simulink model "ur5_v4"  (R2018a)
settings: Solver=VariableStepAuto  StartTime=0.0  StopTime=100.0  MaxStep=2.0  RelTol=1e-3
undefined symbols (not defined in the file): X, Y, Z
libraries: sm_lib x73, nesl_utility x26
(part 3 of 3)

== matlab function ur5_v4/MATLAB Function ==
  data: q1 input; qdot1 input; qddot1 input; tau1 output; q2 input; qdot2 input; qddot2 input; q3 input; qdot3 input; tau2 output; tau3 output; tau4 output; tau5 output; tau6 output; qddot3 input; q4 input; qdot4 input; qddot4 input; q5 input; qdot5 input; qddot5 input; q6 input; qdot6 input; qddot6 input; t input
function [tau1,tau2,tau3,tau4,tau5,tau6] = inverseDynamicsController(q1, qdot1, qddot1, q2, qdot2, qddot2, q3, qdot3, qddot3,q4, qdot4, qddot4,q5, qdot5, qddot5,q6, qdot6, qddot6, t)
    %inverseDynamicsController CTC
    
%     r = 0.7; % m
% %     
% %     % define the gains
% %     kd = eye(6) * 100;
% %     kp = eye(6) * 100;
% % 
% %     % defining the theta vector
% %     q = [q1; q2; q3; q4; q5; q6];
% %     q(1) = mod(q(1),sign(q(1)) * 2*pi);
% %     q(2) = mod(q(2),sign(q(2)) * 2*pi);
% %     q(3) = mod(q(3),sign(q(3)) * 2*pi);
% %     q(4) = mod(q(4),sign(q(4)) * 2*pi);
% %     q(5) = mod(q(5),sign(q(5)) * 2*pi);
% %     q(6) = mod(q(6),sign(q(6)) * 2*pi);
% % 
% %     % defining the theta dot vector
% %     qdot = [qdot1; qdot2; qdot3; qdot4; qdot5; qdot6];
% %     
% %     G = computeG(q);
% %     M = computeM(q);
% %     C = computeC(q, qdot);
% %     
% %     xd = [r * cos(t);...
% %           r * sin(t);...
% %           0.5;...
% %           0;...
% %           0;...
% %           0;...
% %           ];
% %     xdotd = [-r * sin(t);...
% %              r * cos(t);...
% %              0;...
% %              0;...
% %              0;...
% %              0];
% %          
% %     xddotd = [-r * cos(t);...
% %               -r * sin(t);...
% %               0;...
% %               0;...
% %               0;...
% %               0];
% %               
% %     mdl_ur5
% theta = [q1;q2;q3;q4;q5;q6];
% dtheta = [qdot1;qdot2;qdot3;qdot4;qdot5;qdot6];
% %% Dynamics
% Mmat = [ 0.826179504375*cos(2.0*t2 + t3) - 0.0565404972*sin(2.0*t2 + t3) + 1.20557253125*cos(2.0*t2) + 0.0000000000000000019573801614355403439437524183897*cos(t2 + t3) + 0.000000000000000014511003174485468031141763691783*sin(t2 + t3) + 0.826179504375*cos(t3) + 0.000000000000000015722565581023132984666028219267*sin(t2) - 0.0565404972*sin(t3) + 0.374967577853955*cos(2.0*t2 + 2.0*t3) - 0.052183553004*sin(2.0*t2 + 2.0*t3) + 1.6498961438878783371962262793672,                                                    0.015983221960800000770298430129775*cos(t2 + t3) + 0.11849133304875000319532105772424*sin(t2 + t3) + 0.00000000000000010117780855539904452958870603611*cos(t3) + 0.12838449087500000346210694590899*sin(t2) - 0.0000000000000000069242138918179886397619225021053*sin(t3) + 0.00000000000000019510093541407624091515398576369,                           0.015983221960800000770298430129775*cos(t2 + t3) + 0.11849133304875000319532105772424*sin(t2 + t3) + 0.000000000000000050588904277699522264794353018057*cos(t3) - 0.0000000000000000034621069459089943198809612510527*sin(t3) + 0.000000000000000047460881260547746144125949805253;...
%                                                                                                                                   0.015983221960800000770298430129775*cos(t2 + t3) + 0.11849133304875000319532105772424*sin(t2 + t3) + 0.00000000000000010117780855539904452958870603611*cos(t3) + 0.12838449087500000346210694590899*sin(t2) - 0.0000000000000000069242138918179886397619225021053*sin(t3) + 0.00000000000000019510093541407624091515398576369, 3.0976769848028282159067604929052e-33*cos(2.0*t2 + t3) - 2.1199290948066343006048283768305e-34*sin(2.0*t2 + t3) + 4.5201729936265140290864586741331e-33*cos(2.0*t2) + 1.65235900875*cos(t3) - 0.1130809944*sin(t3) + 1.4059032326687268632269500543656e-33*cos(2.0*t2 + 2.0*t3) - 1.9565698527950642456758680724983e-34*sin(2.0*t2 + 2.0*t3) + 4.0105217519862564934991990776325, 1.5488384924014141079533802464526e-33*cos(2.0*t2 + t3) - 1.0599645474033171503024141884152e-34*sin(2.0*t2 + t3) + 0.826179504375*cos(t3) - 0.0565404972*sin(t3) + 1.4059032326687268632269500543656e-33*cos(2.0*t2 + 2.0*t3) - 1.9565698527950642456758680724983e-34*sin(2.0*t2 + 2.0*t3) + 0.77509501177959;...
%                                                                                                                                                                              0.015983221960800000770298430129775*cos(t2 + t3) + 0.11849133304875000319532105772424*sin(t2 + t3) + 0.000000000000000050588904277699522264794353018057*cos(t3) - 0.0000000000000000034621069459089943198809612510527*sin(t3) + 0.000000000000000047460881260547746144125949805253,                                                                     1.5488384924014141079533802464526e-33*cos(2.0*t2 + t3) - 1.0599645474033171503024141884152e-34*sin(2.0*t2 + t3) + 0.826179504375*cos(t3) - 0.0565404972*sin(t3) + 1.4059032326687268632269500543656e-33*cos(2.0*t2 + 2.0*t3) - 1.9565698527950642456758680724983e-34*sin(2.0*t2 + 2.0*t3) + 0.77509501177959,                                                                                                                                                 1.4059032326687268632269500543656e-33*cos(2.0*t2 + 2.0*t3) - 1.9565698527950642456758680724983e-34*sin(2.0*t2 + 2.0*t3) + 0.96104026567958999598344970763719];
%  
% Cmat =[- 0.5*t2_d*(0.1130809944*cos(2.0*t2 + t3)+1.65235900875*sin(2.0*t2 + t3) + 2.4111450625*sin(2.0*t2) - 0.000000000000000014511003174485468031141763691783*cos(t2 + t3) + 0.0000000000000000019573801614355403439437524183897*sin(t2 + t3) - 0.000000000000000015722565581023132984666028219267*cos(t2) + 0.104367106008*cos(2.0*t2 + 2.0*t3) + 0.74993515570791*sin(2.0*t2 + 2.0*t3)) - 0.5*t3_d*(0.0565404972*cos(2.0*t2 + t3) + 0.826179504375*sin(2.0*t2 + t3) - 0.000000000000000014511003174485468031141763691783*cos(t2 + t3) + 0.0000000000000000019573801614355403439437524183897*sin(t2 + t3) + 0.0565404972*cos(t3) + 0.826179504375*sin(t3) + 0.104367106008*cos(2.0*t2 + 2.0*t3) + 0.74993515570791*sin(2.0*t2 + 2.0*t3)),                                                                                                                                          0.0000000000000000072555015872427340155708818458913*cos(t2 + t3) - 0.826179504375*sin(2.0*t2 + t3) - 1.20557253125*sin(2.0*t2) - 0.0565404972*cos(2.0*t2 + t3) - 0.00000000000000000097869008071777017197187620919485*sin(t2 + t3) + 0.0000000000000000078612827905115664923330141096337*cos(t2) - 0.052183553004*cos(2.0*t2 + 2.0*t3) - 0.374967577853955*sin(2.0*t2 + 2.0*t3) - 0.5*t3_d*(0.031966443921600001540596860259551*sin(t2 + t3) - 0.23698266609750000639064211544848*cos(t2 + t3) + 0.0000000000000000069242138918179886397619225021053*cos(t3) + 0.00000000000000010117780855539904452958870603611*sin(t3)) + 0.5*t2_d*(0.23698266609750000639064211544848*cos(t2 + t3) - 0.031966443921600001540596860259551*sin(t2 + t3) + 0.25676898175000000692421389181799*cos(t2)),                                                                                                                                 0.0000000000000000072555015872427340155708818458913*cos(t2 + t3) - 0.4130897521875*sin(2.0*t2 + t3) - 0.0282702486*cos(2.0*t2 + t3) - 0.00000000000000000097869008071777017197187620919485*sin(t2 + t3) - 0.0282702486*cos(t3) - 0.4130897521875*sin(t3) - 0.052183553004*cos(2.0*t2 + 2.0*t3) - 0.374967577853955*sin(2.0*t2 + 2.0*t3) - 0.5*t2_d*(0.031966443921600001540596860259551*sin(t2 + t3) - 0.23698266609750000639064211544848*cos(t2 + t3) + 0.0000000000000000069242138918179886397619225021053*cos(t3) + 0.00000000000000010117780855539904452958870603611*sin(t3)) - 0.5*t3_d*(0.031966443921600001540596860259551*sin(t2 + t3) - 0.23698266609750000639064211544848*cos(t2 + t3) + 0.0000000000000000069242138918179886397619225021053*cos(t3) + 0.00000000000000010117780855539904452958870603611*sin(t3));...
%                                                                                                                                                                                                               0.5*t1_d*(0.1130809944*cos(2.0*t2 + t3) + 1.65235900875*sin(2.0*t2 + t3) + 2.4111450625*sin(2.0*t2) - 0.000000000000000014511003174485468031141763691783*cos(t2 + t3) + 0.0000000000000000019573801614355403439437524183897*sin(t2 + t3) - 0.000000000000000015722565581023132984666028219267*cos(t2) + 0.104367106008*cos(2.0*t2 + 2.0*t3) + 0.74993515570791*sin(2.0*t2 + 2.0*t3)) - 0.5*t3_d*(0.0000000000000000069242138918179886397619225021053*cos(t3) + 0.00000000000000010117780855539904452958870603611*sin(t3)), 0.059245666524375001597660528862121*cos(t2 + t3) - 0.0079916109804000003851492150648877*sin(t2 + t3) + 0.064192245437500001731053472954497*cos(t2) - 0.5*t1_d*(0.11849133304875000319532105772424*cos(t2 + t3) - 0.015983221960800000770298430129775*sin(t2 + t3) + 0.12838449087500000346210694590899*cos(t2)) - 0.5*t2_d*(4.239858189613268601209656753661e-34*cos(2.0*t2 + t3) + 6.1953539696056564318135209858103e-33*sin(2.0*t2 + t3) + 9.0403459872530280581729173482661e-33*sin(2.0*t2) + 3.9131397055901284913517361449965e-34*cos(2.0*t2 + 2.0*t3) + 2.8118064653374537264539001087311e-33*sin(2.0*t2 + 2.0*t3)) - 0.5*t3_d*(2.1199290948066343006048283768305e-34*cos(2.0*t2 + t3) + 3.0976769848028282159067604929052e-33*sin(2.0*t2 + t3) + 0.1130809944*cos(t3) + 1.65235900875*sin(t3) + 3.9131397055901284913517361449965e-34*cos(2.0*t2 + 2.0*t3) + 2.8118064653374537264539001087311e-33*sin(2.0*t2 + 2.0*t3)), 0.059245666524375001597660528862121*cos(t2 + t3) - 0.0079916109804000003851492150648877*sin(t2 + t3) - 0.0000000000000000034621069459089943198809612510527*cos(t3) - 0.000000000000000050588904277699522264794353018057*sin(t3) - 0.5*t1_d*(0.11849133304875000319532105772424*cos(t2 + t3) - 0.015983221960800000770298430129775*sin(t2 + t3)) - 0.5*t2_d*(2.1199290948066343006048283768305e-34*cos(2.0*t2 + t3) + 3.0976769848028282159067604929052e-33*sin(2.0*t2 + t3) + 0.1130809944*cos(t3) + 1.65235900875*sin(t3) + 3.9131397055901284913517361449965e-34*cos(2.0*t2 + 2.0*t3) + 2.8118064653374537264539001087311e-33*sin(2.0*t2 + 2.0*t3)) - 0.5*t3_d*(2.1199290948066343006048283768305e-34*cos(2.0*t2 + t3) + 3.0976769848028282159067604929052e-33*sin(2.0*t2 + t3) + 0.1130809944*cos(t3) + 1.65235900875*sin(t3) + 3.9131397055901284913517361449965e-34*cos(2.0*t2 + 2.0*t3) + 2.8118064653374537264539001087311e-33*sin(2.0*t2 + 2.0*t3));...
%                                                                                                                                                                                                                                                      0.5*t2_d*(0.0000000000000000069242138918179886397619225021053*cos(t3) + 0.00000000000000010117780855539904452958870603611*sin(t3)) + 0.5*t1_d*(0.0565404972*cos(2.0*t2 + t3) + 0.826179504375*sin(2.0*t2 + t3) - 0.000000000000000014511003174485468031141763691783*cos(t2 + t3) + 0.0000000000000000019573801614355403439437524183897*sin(t2 + t3) + 0.0565404972*cos(t3) + 0.826179504375*sin(t3) + 0.104367106008*cos(2.0*t2 + 2.0*t3) + 0.74993515570791*sin(2.0*t2 + 2.0*t3)),                                                                                                                                       0.059245666524375001597660528862121*cos(t2 + t3) - 0.0079916109804000003851492150648877*sin(t2 + t3) + 0.5*t1_d*(0.015983221960800000770298430129775*sin(t2 + t3) - 0.11849133304875000319532105772424*cos(t2 + t3) + 0.0000000000000000069242138918179886397619225021053*cos(t3) + 0.00000000000000010117780855539904452958870603611*sin(t3)) - 0.5*t3_d*(3.9131397055901284913517361449965e-34*cos(2.0*t2 + 2.0*t3) + 2.8118064653374537264539001087311e-33*sin(2.0*t2 + 2.0*t3)) - 0.5*t2_d*(2.1199290948066343006048283768305e-34*cos(2.0*t2 + t3) + 3.0976769848028282159067604929052e-33*sin(2.0*t2 + t3) - 0.1130809944*cos(t3) - 1.65235900875*sin(t3) + 3.9131397055901284913517361449965e-34*cos(2.0*t2 + 2.0*t3) + 2.8118064653374537264539001087311e-33*sin(2.0*t2 + 2.0*t3)),                                                                                                                                                                                                        0.059245666524375001597660528862121*cos(t2 + t3) - 0.0079916109804000003851492150648877*sin(t2 + t3) - 0.0000000000000000017310534729544971599404806255263*cos(t3) - 0.000000000000000025294452138849761132397176509029*sin(t3) + 0.5*t1_d*(0.015983221960800000770298430129775*sin(t2 + t3) - 0.11849133304875000319532105772424*cos(t2 + t3) + 0.0000000000000000034621069459089943198809612510527*cos(t3) + 0.000000000000000050588904277699522264794353018057*sin(t3)) - 0.5*t2_d*(3.9131397055901284913517361449965e-34*cos(2.0*t2 + 2.0*t3) + 2.8118064653374537264539001087311e-33*sin(2.0*t2 + 2.0*t3)) - 0.5*t3_d*(3.9131397055901284913517361449965e-34*cos(2.0*t2 + 2.0*t3) + 2.8118064653374537264539001087311e-33*sin(2.0*t2 + 2.0*t3))];
% Gmat = g*[1.5200799240000000184971359776743 - 1.943951775*sin(t2 + t3) - 5.6732825*sin(t2) - 0.133036464*cos(t2 + t3);...
%  1.5200799240000000184971359776743 - 1.943951775*sin(t2 + t3) - 5.6732825*sin(t2) - 0.133036464*cos(t2 + t3);...
%  1.5200799240000000184971359776743 - 1.943951775*sin(t2 + t3) - 5.6732825*sin(t2) - 0.133036464*cos(t2 + t3)];
% invM = inv(Mmat);
% %% Jacobian
% J = [ 0.19145000000000000579013006636869*cos(t1) + 0.39225*cos(t3)*(0.00000000000000006123233995736766035868820147292*cos(t1)*sin(t2) + cos(t2)*sin(t1)) + 0.000000000000000026023744481881255652442485625991*cos(t1)*sin(t2) + 0.425*cos(t2)*sin(t1) - 0.09456*sin(t3)*(0.00000000000000006123233995736766035868820147292*cos(t1)*sin(t2) + cos(t2)*sin(t1)) + 0.09456*cos(t3)*(0.00000000000000006123233995736766035868820147292*cos(t1)*cos(t2) - 1.0*sin(t1)*sin(t2)) + 0.39225*sin(t3)*(0.00000000000000006123233995736766035868820147292*cos(t1)*cos(t2) - 1.0*sin(t1)*sin(t2)),         0.09456*cos(t3)*(cos(t1)*cos(t2) - 0.00000000000000006123233995736766035868820147292*sin(t1)*sin(t2)) + 0.39225*cos(t3)*(cos(t1)*sin(t2) + 0.00000000000000006123233995736766035868820147292*cos(t2)*sin(t1)) + 0.425*cos(t1)*sin(t2) + 0.000000000000000026023744481881255652442485625991*cos(t2)*sin(t1) + 0.39225*sin(t3)*(cos(t1)*cos(t2) - 0.00000000000000006123233995736766035868820147292*sin(t1)*sin(t2)) - 0.09456*sin(t3)*(cos(t1)*sin(t2) + 0.00000000000000006123233995736766035868820147292*cos(t2)*sin(t1)),         0.09456*cos(t3)*(cos(t1)*cos(t2) - 0.00000000000000006123233995736766035868820147292*sin(t1)*sin(t2)) + 0.39225*cos(t3)*(cos(t1)*sin(t2) + 0.00000000000000006123233995736766035868820147292*cos(t2)*sin(t1)) + 0.39225*sin(t3)*(cos(t1)*cos(t2) - 0.00000000000000006123233995736766035868820147292*sin(t1)*sin(t2)) - 0.09456*sin(t3)*(cos(t1)*sin(t2) + 0.00000000000000006123233995736766035868820147292*cos(t2)*sin(t1));...
%          0.19145000000000000579013006636869*sin(t1) - 0.425*cos(t1)*cos(t2) - 0.39225*cos(t3)*(cos(t1)*cos(t2) - 0.00000000000000006123233995736766035868820147292*sin(t1)*sin(t2)) + 0.09456*cos(t3)*(cos(t1)*sin(t2) + 0.00000000000000006123233995736766035868820147292*cos(t2)*sin(t1)) + 0.09456*sin(t3)*(cos(t1)*cos(t2) - 0.00000000000000006123233995736766035868820147292*sin(t1)*sin(t2)) + 0.39225*sin(t3)*(cos(t1)*sin(t2) + 0.00000000000000006123233995736766035868820147292*cos(t2)*sin(t1)) + 0.000000000000000026023744481881255652442485625991*sin(t1)*sin(t2), 0.09456*cos(t3)*(0.00000000000000006123233995736766035868820147292*cos(t1)*sin(t2) + cos(t2)*sin(t1)) - 0.000000000000000026023744481881255652442485625991*cos(t1)*cos(t2) + 0.39225*sin(t3)*(0.00000000000000006123233995736766035868820147292*cos(t1)*sin(t2) + cos(t2)*sin(t1)) + 0.425*sin(t1)*sin(t2) - 0.39225*cos(t3)*(0.00000000000000006123233995736766035868820147292*cos(t1)*cos(t2) - 1.0*sin(t1)*sin(t2)) + 0.09456*sin(t3)*(0.00000000000000006123233995736766035868820147292*cos(t1)*cos(t2) - 1.0*sin(t1)*sin(t2)), 0.09456*cos(t3)*(0.00000000000000006123233995736766035868820147292*cos(t1)*sin(t2) + cos(t2)*sin(t1)) + 0.39225*sin(t3)*(0.00000000000000006123233995736766035868820147292*cos(t1)*sin(t2) + cos(t2)*sin(t1)) - 0.39225*cos(t3)*(0.00000000000000006123233995736766035868820147292*cos(t1)*cos(t2) - 1.0*sin(t1)*sin(t2)) + 0.09456*sin(t3)*(0.00000000000000006123233995736766035868820147292*cos(t1)*cos(t2) - 1.0*sin(t1)*sin(t2));...
%                                                                                                                                                                                                                                                                                                                                                                                                                                                                                                                                                                                0,                                                                                                                                                                                                                                                                                                                                                                                                              0.09456*cos(t2)*sin(t3) - 0.39225*cos(t2)*cos(t3) - 0.425*cos(t2) + 0.09456*cos(t3)*sin(t2) + 0.39225*sin(t2)*sin(t3),                                                                                                                                                                                                                                                                                                                                 0.09456*cos(t2)*sin(t3) - 0.39225*cos(t2)*cos(t3) + 0.09456*cos(t3)*sin(t2) + 0.39225*sin(t2)*sin(t3)];
% Jdot = [ 0.39225*cos(t3)*(t1_d*cos(t1)*cos(t2) + 0.00000000000000006123233995736766035868820147292*t2_d*cos(t1)*cos(t2) - 0.00000000000000006123233995736766035868820147292*t1_d*sin(t1)*sin(t2) - 1.0*t2_d*sin(t1)*sin(t2)) - 0.19145000000000000579013006636869*t1_d*sin(t1) - 0.09456*sin(t3)*(t1_d*cos(t1)*cos(t2) + 0.00000000000000006123233995736766035868820147292*t2_d*cos(t1)*cos(t2) - 0.00000000000000006123233995736766035868820147292*t1_d*sin(t1)*sin(t2) - 1.0*t2_d*sin(t1)*sin(t2)) - 0.09456*cos(t3)*(1.0*t1_d*cos(t1)*sin(t2) + 0.00000000000000006123233995736766035868820147292*t1_d*cos(t2)*sin(t1) + 0.00000000000000006123233995736766035868820147292*t2_d*cos(t1)*sin(t2) + 1.0*t2_d*cos(t2)*sin(t1)) - 0.39225*sin(t3)*(1.0*t1_d*cos(t1)*sin(t2) + 0.00000000000000006123233995736766035868820147292*t1_d*cos(t2)*sin(t1) + 0.00000000000000006123233995736766035868820147292*t2_d*cos(t1)*sin(t2) + 1.0*t2_d*cos(t2)*sin(t1)) + 0.425*t1_d*cos(t1)*cos(t2) + 0.000000000000000026023744481881255652442485625991*t2_d*cos(t1)*cos(t2) - 0.09456*t3_d*cos(t3)*(0.00000000000000006123233995736766035868820147292*cos(t1)*sin(t2) + cos(t2)*sin(t1)) - 0.39225*t3_d*sin(t3)*(0.00000000000000006123233995736766035868820147292*cos(t1)*sin(t2) + cos(t2)*sin(t1)) - 0.000000000000000026023744481881255652442485625991*t1_d*sin(t1)*sin(t2) - 0.425*t2_d*sin(t1)*sin(t2) + 0.39225*t3_d*cos(t3)*(0.00000000000000006123233995736766035868820147292*cos(t1)*cos(t2) - 1.0*sin(t1)*sin(t2)) - 0.09456*t3_d*sin(t3)*(0.00000000000000006123233995736766035868820147292*cos(t1)*cos(t2) - 1.0*sin(t1)*sin(t2)),                         0.39225*cos(t3)*(0.00000000000000006123233995736766035868820147292*t1_d*cos(t1)*cos(t2) + t2_d*cos(t1)*cos(t2) - 1.0*t1_d*sin(t1)*sin(t2) - 0.00000000000000006123233995736766035868820147292*t2_d*sin(t1)*sin(t2)) - 0.39225*sin(t3)*(0.00000000000000006123233995736766035868820147292*t1_d*cos(t1)*sin(t2) + t1_d*cos(t2)*sin(t1) + t2_d*cos(t1)*sin(t2) + 0.00000000000000006123233995736766035868820147292*t2_d*cos(t2)*sin(t1)) - 0.09456*cos(t3)*(0.00000000000000006123233995736766035868820147292*t1_d*cos(t1)*sin(t2) + t1_d*cos(t2)*sin(t1) + t2_d*cos(t1)*sin(t2) + 0.00000000000000006123233995736766035868820147292*t2_d*cos(t2)*sin(t1)) - 0.09456*sin(t3)*(0.00000000000000006123233995736766035868820147292*t1_d*cos(t1)*cos(t2) + t2_d*cos(t1)*cos(t2) - 1.0*t1_d*sin(t1)*sin(t2) - 0.00000000000000006123233995736766035868820147292*t2_d*sin(t1)*sin(t2)) + 0.000000000000000026023744481881255652442485625991*t1_d*cos(t1)*cos(t2) + 0.425*t2_d*cos(t1)*cos(t2) + 0.39225*t3_d*cos(t3)*(cos(t1)*cos(t2) - 0.00000000000000006123233995736766035868820147292*sin(t1)*sin(t2)) - 0.09456*t3_d*cos(t3)*(cos(t1)*sin(t2) + 0.00000000000000006123233995736766035868820147292*cos(t2)*sin(t1)) - 0.09456*t3_d*sin(t3)*(cos(t1)*cos(t2) - 0.00000000000000006123233995736766035868820147292*sin(t1)*sin(t2)) - 0.39225*t3_d*sin(t3)*(cos(t1)*sin(t2) + 0.00000000000000006123233995736766035868820147292*cos(t2)*sin(t1)) - 0.425*t1_d*sin(t1)*sin(t2) - 0.000000000000000026023744481881255652442485625991*t2_d*sin(t1)*sin(t2),                         0.39225*cos(t3)*(0.00000000000000006123233995736766035868820147292*t1_d*cos(t1)*cos(t2) + t2_d*cos(t1)*cos(t2) - 1.0*t1_d*sin(t1)*sin(t2) - 0.00000000000000006123233995736766035868820147292*t2_d*sin(t1)*sin(t2)) - 0.39225*sin(t3)*(0.00000000000000006123233995736766035868820147292*t1_d*cos(t1)*sin(t2) + t1_d*cos(t2)*sin(t1) + t2_d*cos(t1)*sin(t2) + 0.00000000000000006123233995736766035868820147292*t2_d*cos(t2)*sin(t1)) - 0.09456*cos(t3)*(0.00000000000000006123233995736766035868820147292*t1_d*cos(t1)*sin(t2) + t1_d*cos(t2)*sin(t1) + t2_d*cos(t1)*sin(t2) + 0.00000000000000006123233995736766035868820147292*t2_d*cos(t2)*sin(t1)) - 0.09456*sin(t3)*(0.00000000000000006123233995736766035868820147292*t1_d*cos(t1)*cos(t2) + t2_d*cos(t1)*cos(t2) - 1.0*t1_d*sin(t1)*sin(t2) - 0.00000000000000006123233995736766035868820147292*t2_d*sin(t1)*sin(t2)) + 0.39225*t3_d*cos(t3)*(cos(t1)*cos(t2) - 0.00000000000000006123233995736766035868820147292*sin(t1)*sin(t2)) - 0.09456*t3_d*cos(t3)*(cos(t1)*sin(t2) + 0.00000000000000006123233995736766035868820147292*cos(t2)*sin(t1)) - 0.09456*t3_d*sin(t3)*(cos(t1)*cos(t2) - 0.00000000000000006123233995736766035868820147292*sin(t1)*sin(t2)) - 0.39225*t3_d*sin(t3)*(cos(t1)*sin(t2) + 0.00000000000000006123233995736766035868820147292*cos(t2)*sin(t1));...
%                          0.39225*cos(t3)*(0.00000000000000006123233995736766035868820147292*t1_d*cos(t1)*sin(t2) + t1_d*cos(t2)*sin(t1) + t2_d*cos(t1)*sin(t2) + 0.00000000000000006123233995736766035868820147292*t2_d*cos(t2)*sin(t1)) - 0.09456*sin(t3)*(0.00000000000000006123233995736766035868820147292*t1_d*cos(t1)*sin(t2) + t1_d*cos(t2)*sin(t1) + t2_d*cos(t1)*sin(t2) + 0.00000000000000006123233995736766035868820147292*t2_d*cos(t2)*sin(t1)) + 0.19145000000000000579013006636869*t1_d*cos(t1) + 0.09456*cos(t3)*(0.00000000000000006123233995736766035868820147292*t1_d*cos(t1)*cos(t2) + t2_d*cos(t1)*cos(t2) - 1.0*t1_d*sin(t1)*sin(t2) - 0.00000000000000006123233995736766035868820147292*t2_d*sin(t1)*sin(t2)) + 0.39225*sin(t3)*(0.00000000000000006123233995736766035868820147292*t1_d*cos(t1)*cos(t2) + t2_d*cos(t1)*cos(t2) - 1.0*t1_d*sin(t1)*sin(t2) - 0.00000000000000006123233995736766035868820147292*t2_d*sin(t1)*sin(t2)) + 0.09456*t3_d*cos(t3)*(cos(t1)*cos(t2) - 0.00000000000000006123233995736766035868820147292*sin(t1)*sin(t2)) + 0.39225*t3_d*cos(t3)*(cos(t1)*sin(t2) + 0.00000000000000006123233995736766035868820147292*cos(t2)*sin(t1)) + 0.000000000000000026023744481881255652442485625991*t1_d*cos(t1)*sin(t2) + 0.425*t1_d*cos(t2)*sin(t1) + 0.425*t2_d*cos(t1)*sin(t2) + 0.000000000000000026023744481881255652442485625991*t2_d*cos(t2)*sin(t1) + 0.39225*t3_d*sin(t3)*(cos(t1)*cos(t2) - 0.00000000000000006123233995736766035868820147292*sin(t1)*sin(t2)) - 0.09456*t3_d*sin(t3)*(cos(t1)*sin(t2) + 0.00000000000000006123233995736766035868820147292*cos(t2)*sin(t1)), 0.09456*cos(t3)*(t1_d*cos(t1)*cos(t2) + 0.00000000000000006123233995736766035868820147292*t2_d*cos(t1)*cos(t2) - 0.00000000000000006123233995736766035868820147292*t1_d*sin(t1)*sin(t2) - 1.0*t2_d*sin(t1)*sin(t2)) + 0.39225*sin(t3)*(t1_d*cos(t1)*cos(t2) + 0.00000000000000006123233995736766035868820147292*t2_d*cos(t1)*cos(t2) - 0.00000000000000006123233995736766035868820147292*t1_d*sin(t1)*sin(t2) - 1.0*t2_d*sin(t1)*sin(t2)) + 0.39225*cos(t3)*(1.0*t1_d*cos(t1)*sin(t2) + 0.00000000000000006123233995736766035868820147292*t1_d*cos(t2)*sin(t1) + 0.00000000000000006123233995736766035868820147292*t2_d*cos(t1)*sin(t2) + 1.0*t2_d*cos(t2)*sin(t1)) - 0.09456*sin(t3)*(1.0*t1_d*cos(t1)*sin(t2) + 0.00000000000000006123233995736766035868820147292*t1_d*cos(t2)*sin(t1) + 0.00000000000000006123233995736766035868820147292*t2_d*cos(t1)*sin(t2) + 1.0*t2_d*cos(t2)*sin(t1)) + 0.39225*t3_d*cos(t3)*(0.00000000000000006123233995736766035868820147292*cos(t1)*sin(t2) + cos(t2)*sin(t1)) + 0.425*t1_d*cos(t1)*sin(t2) + 0.000000000000000026023744481881255652442485625991*t1_d*cos(t2)*sin(t1) + 0.000000000000000026023744481881255652442485625991*t2_d*cos(t1)*sin(t2) + 0.425*t2_d*cos(t2)*sin(t1) - 0.09456*t3_d*sin(t3)*(0.00000000000000006123233995736766035868820147292*cos(t1)*sin(t2) + cos(t2)*sin(t1)) + 0.09456*t3_d*cos(t3)*(0.00000000000000006123233995736766035868820147292*cos(t1)*cos(t2) - 1.0*sin(t1)*sin(t2)) + 0.39225*t3_d*sin(t3)*(0.00000000000000006123233995736766035868820147292*cos(t1)*cos(t2) - 1.0*sin(t1)*sin(t2)), 0.09456*cos(t3)*(t1_d*cos(t1)*cos(t2) + 0.00000000000000006123233995736766035868820147292*t2_d*cos(t1)*cos(t2) - 0.00000000000000006123233995736766035868820147292*t1_d*sin(t1)*sin(t2) - 1.0*t2_d*sin(t1)*sin(t2)) + 0.39225*sin(t3)*(t1_d*cos(t1)*cos(t2) + 0.00000000000000006123233995736766035868820147292*t2_d*cos(t1)*cos(t2) - 0.00000000000000006123233995736766035868820147292*t1_d*sin(t1)*sin(t2) - 1.0*t2_d*sin(t1)*sin(t2)) + 0.39225*cos(t3)*(1.0*t1_d*cos(t1)*sin(t2) + 0.00000000000000006123233995736766035868820147292*t1_d*cos(t2)*sin(t1) + 0.00000000000000006123233995736766035868820147292*t2_d*cos(t1)*sin(t2) + 1.0*t2_d*cos(t2)*sin(t1)) - 0.09456*sin(t3)*(1.0*t1_d*cos(t1)*sin(t2) + 0.00000000000000006123233995736766035868820147292*t1_d*cos(t2)*sin(t1) + 0.00000000000000006123233995736766035868820147292*t2_d*cos(t1)*sin(t2) + 1.0*t2_d*cos(t2)*sin(t1)) + 0.39225*t3_d*cos(t3)*(0.00000000000000006123233995736766035868820147292*cos(t1)*sin(t2) + cos(t2)*sin(t1)) - 0.09456*t3_d*sin(t3)*(0.00000000000000006123233995736766035868820147292*cos(t1)*sin(t2) + cos(t2)*sin(t1)) + 0.09456*t3_d*cos(t3)*(0.00000000000000006123233995736766035868820147292*cos(t1)*cos(t2) - 1.0*sin(t1)*sin(t2)) + 0.39225*t3_d*sin(t3)*(0.00000000000000006123233995736766035868820147292*cos(t1)*cos(t2) - 1.0*sin(t1)*sin(t2));...
%                                                                                                                                                                                                                                                                                                                                                                                                                                                                                                                                                                                                                                                                                                                                                                                                                                                                                                                                                                                                                                                                                                                                                                                                                                                                                                                                                                                                                                                                                                                                                                                                                          0,                                                                                                                                                                                                                                                                                                                                                                                                                                                                                                                                                                                                                                                                                                                                                                                                                                                                                                                                                                                                                                                                                                                                                                                                                                                                                              0.425*t2_d*sin(t2) + 0.09456*t2_d*cos(t2)*cos(t3) + 0.09456*t3_d*cos(t2)*cos(t3) + 0.39225*t2_d*cos(t2)*sin(t3) + 0.39225*t2_d*cos(t3)*sin(t2) + 0.39225*t3_d*cos(t2)*sin(t3) + 0.39225*t3_d*cos(t3)*sin(t2) - 0.09456*t2_d*sin(t2)*sin(t3) - 0.09456*t3_d*sin(t2)*sin(t3),                                                                                                                                                                                                                                                                                                                                                                                                                                                                                                                                                                                                                                                                                                                                                                                                                                                                                                                                                                                                                                                                                                     0.09456*t2_d*cos(t2)*cos(t3) + 0.09456*t3_d*cos(t2)*cos(t3) + 0.39225*t2_d*cos(t2)*sin(t3) + 0.39225*t2_d*cos(t3)*sin(t2) + 0.39225*t3_d*cos(t2)*sin(t3) + 0.39225*t3_d*cos(t3)*sin(t2) - 0.09456*t2_d*sin(t2)*sin(t3) - 0.09456*t3_d*sin(t2)*sin(t3)];
% 
% T = fk_ur5(t1,t2,t3);
% x = [T(1,4);T(2,4);T(3,4)];
% xdot = J*dtheta;
% x_d = [0.2*sin(0.01*t)-0.4;0.2*cos(0.01*t)-0.4;-0.1];
% dx_d = 0.01*[0.2*cos(0.01*t);-0.2*sin(0.01*t);0];
% ddx_d = 0.01^2*[-0.2*sin(0.01*t);-0.2*cos(0.01*t);0];
% % x_d = [-0.1904;-0.0201;0.1107];
% % dx_d = [0;0;0];
% % ddx_d = [0;0;0];
% % x_d =  [-0.6905*(t/100)-0.6882*(1-t/100);-0.3348*(t/100)-0.3952*(1-t/100);-0.2351];
% % dx_d =  1.0e-03 *[-0.0230;0.6040;0];
% % ddx_d = [0;0;0];
% x-x_d
% ddx = ddx_d - Kp*(x-x_d)-Kd*(xdot-dx_d);
% Torque = Mmat*(inv(J)*ddx - Jdot*dtheta)+ Cmat*dtheta +Gmat;
% dq = [dtheta; invM*(Torque- Gmat)-invM*Cmat*dtheta];
Torque = [0;0;0;0;0;0];
   
tau1 = Torque(1);
tau2 = Torque(2);
tau3 = Torque(3);
tau4 = Torque(4);
tau5 = Torque(5);
tau6 = Torque(6);
